simulink model "sim1"  (R2015b)
settings: Solver=VariableStepAuto  StartTime=0.0  StopTime=10.0  RelTol=1e-3
settings Model: Creator=ovi  LastModifiedBy=ovi

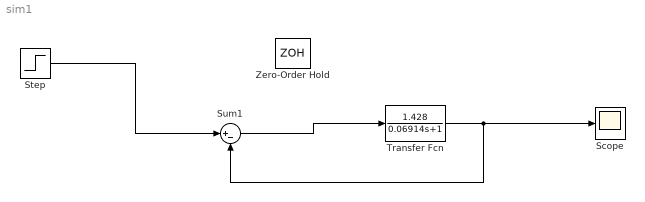
== system sim1 ==
  Scope : Scope
  Step : Step  SampleTime=0
  Sum1 : Sum  Inputs=|+-
  Transfer Fcn : TransferFcn  Numerator=[1.428]  Denominator=[0.06914 1]
  Zero-Order Hold : ZeroOrderHold
  wires:
  Transfer Fcn/1 -> Sum1/2, Scope/1
  Step/1 -> Sum1/1
  Sum1/1 -> Transfer Fcn/1
